simulink model "swapna_1"  (R2017a)
settings: Solver=VariableStepAuto  StartTime=0.0  StopTime=0.5  MaxStep=1e-4  RelTol=1e-3
libraries: powerlib x15
settings Model: Creator=Gali  LastModifiedBy=Gali

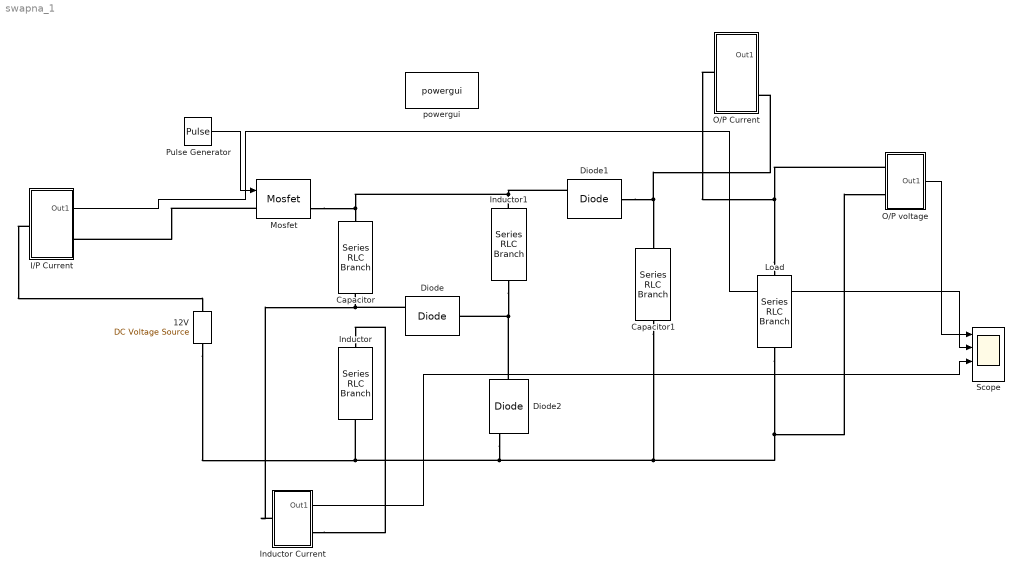
== system swapna_1 ==
  12V : powerlib/Electrical Sources/DC Voltage Source  Amplitude=12  Measurements=None
  Capacitor : powerlib/Elements/Series RLC Branch  LConnTagsString=__new0  RConnTagsString=__new0  BranchType=C  Resistance=1  Inductance=1e-3  SetiL0=off  InitialCurrent=0  Capacitance=47e-6  Setx0=off  InitialVoltage=0  Measurements=None
  Capacitor1 : powerlib/Elements/Series RLC Branch  LConnTagsString=__new0  RConnTagsString=__new0  BranchType=C  Resistance=1  Inductance=1e-3  SetiL0=off  InitialCurrent=0  Capacitance=270e-6  Setx0=off  InitialVoltage=0  Measurements=None
  Diode : powerlib/Power Electronics/Diode  Ron=0.001  Lon=0  Vf=0.8  IC=0  UseSnubber=0  Rs=500  Cs=250e-9  Measurements=on
  Diode1 : powerlib/Power Electronics/Diode  Ron=0.001  Lon=0  Vf=0.8  IC=0  UseSnubber=0  Rs=500  Cs=250e-9  Measurements=on
  Diode2 : powerlib/Power Electronics/Diode  Ron=0.001  Lon=0  Vf=0.8  IC=0  UseSnubber=0  Rs=500  Cs=250e-9  Measurements=on
  I/P Current : Subsystem
  Inductor : powerlib/Elements/Series RLC Branch  LConnTagsString=__new0  RConnTagsString=__new0  BranchType=L  Resistance=1  Inductance=1e-3  SetiL0=off  InitialCurrent=0  Capacitance=1e-6  Setx0=off  InitialVoltage=0  Measurements=None
  Inductor Current : Subsystem
  Inductor1 : powerlib/Elements/Series RLC Branch  LConnTagsString=__new0  RConnTagsString=__new0  BranchType=L  Resistance=1  Inductance=1e-3  SetiL0=off  InitialCurrent=0  Capacitance=1e-6  Setx0=off  InitialVoltage=0  Measurements=None
  Load : powerlib/Elements/Series RLC Branch  LConnTagsString=__new0  RConnTagsString=__new0  BranchType=R  Resistance=47  Inductance=1e-3  SetiL0=off  InitialCurrent=0  Capacitance=220e-6  Setx0=off  InitialVoltage=0  Measurements=None
  Mosfet : powerlib/Power Electronics/Mosfet  Ron=0.28  Lon=0  Rd=0.01  Vfd=0  IC=0  Rs=1e5  Cs=inf  Measurements=on
  O/P Current : Subsystem
  O/P voltage : Subsystem
  Pulse Generator : DiscretePulseGenerator  PulseType=Time based  Period=1/32000  PulseWidth=62.2
  Scope : Scope  NumInputPorts=4
  powergui : powerlib/powergui  Priority=1  SimulationMode=Continuous  SampleTime=50e-6  frequency=60  Iterations=50  frequencyindice=0  Pbase=100e6  ErrMax=1e-4  UnitsV=kV  UnitsW=MW  buscounter=0  FunctionMessages=off  echomessages=off  EnableUseOfTLC=off  CurrentSourceSwitches=off  DisableSnubberDevices=off  DisableRonSwitches=off  DisableVfSwitches=off  DisplayEquations=off  SolverType=Tustin/Backward Euler (TBE)  Interpol=off  ExternalGateDelay=off  methode=off  Ts=100  x0status=blocks  SPID=on  SwTol=0  HookPort=off  RestoreLinks=warning  ResistiveCurrentMeasurement=off  Frange=[0:2:500]  Ylog=off  Xlog=on  ShowGrid=off  save=off  variable=ZData  structure=0  ZoomFFT=off  StartTime=0.0  cycles=1  DisplayStyle=1  fundamental=60  FreqAxis=off  MaxFrequency=1000  frequencyindicesteady=1  RmsSteady=1  display=off
  wires:
  Pulse Generator/1 -> Mosfet/1
  I/P Current/1(Out1) -> Scope/2
  O/P voltage/1(Out1) -> Scope/1
  Inductor Current/1(Out1) -> Scope/3
  connections:
  Load/RConn1 -- O/P voltage/LConn2 -- Capacitor1/LConn1 -- Diode2/RConn1 -- 12V/LConn1 -- Inductor/RConn1
  Capacitor/RConn1 -- Diode1/RConn1 -- Inductor1/LConn1 -- Mosfet/RConn1
  Inductor1/RConn1 -- Diode2/LConn1 -- Diode/LConn1
  Diode1/LConn1 -- O/P Current/RConn1 -- Capacitor1/RConn1
  Mosfet/LConn1 -- I/P Current/RConn1
  I/P Current/LConn1 -- 12V/RConn1
  Load/LConn1 -- O/P voltage/LConn1 -- O/P Current/LConn1
  Capacitor/LConn1 -- Inductor Current/LConn1 -- Diode/RConn1
  Inductor Current/RConn1 -- Inductor/LConn1

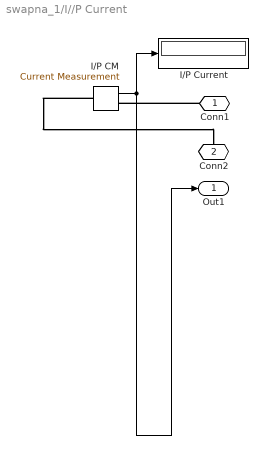
== system swapna_1/I//P Current ==
  I/P CM : powerlib/Measurements/Current Measurement  PhasorSimulation=off  OutputType=Complex  PSBequivalent=0
  I/P Current : Display
  Conn1 : PMIOPort  Port=1  Side=Right
  Conn2 : PMIOPort  Port=2  Side=Left
  Out1 : Outport
  wires:
  I/P CM/1 -> Out1/1, I/P Current/1
  connections:
  Conn1/RConn1 -- I/P CM/RConn1
  I/P CM/LConn1 -- Conn2/RConn1

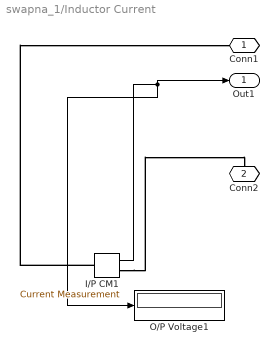
== system swapna_1/Inductor Current ==
  I/P CM1 : powerlib/Measurements/Current Measurement  PhasorSimulation=off  OutputType=Complex  PSBequivalent=0
  O/P Voltage1 : Display
  Conn1 : PMIOPort  Port=1  Side=Left
  Conn2 : PMIOPort  Port=2  Side=Right
  Out1 : Outport
  wires:
  I/P CM1/1 -> Out1/1, O/P Voltage1/1
  connections:
  I/P CM1/LConn1 -- Conn1/RConn1
  I/P CM1/RConn1 -- Conn2/RConn1

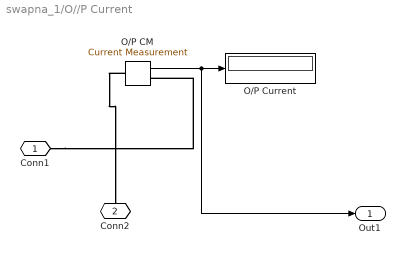
== system swapna_1/O//P Current ==
  O/P CM : powerlib/Measurements/Current Measurement  PhasorSimulation=off  OutputType=Complex  PSBequivalent=0
  O/P Current : Display
  Conn1 : PMIOPort  Port=1  Side=Right
  Conn2 : PMIOPort  Port=2  Side=Left
  Out1 : Outport
  wires:
  O/P CM/1 -> Out1/1, O/P Current/1
  connections:
  Conn1/RConn1 -- O/P CM/RConn1
  O/P CM/LConn1 -- Conn2/RConn1

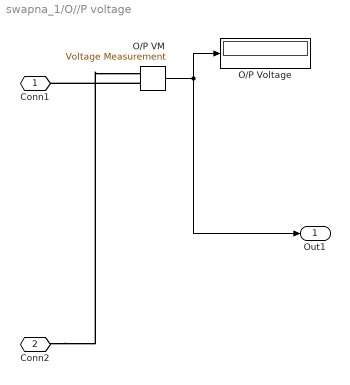
== system swapna_1/O//P voltage ==
  O/P VM : powerlib/Measurements/Voltage Measurement  PhasorSimulation=off  OutputType=Complex  PSBequivalent=0
  O/P Voltage : Display
  Conn1 : PMIOPort  Port=1  Side=Left
  Conn2 : PMIOPort  Port=2  Side=Left
  Out1 : Outport
  wires:
  O/P VM/1 -> Out1/1, O/P Voltage/1
  connections:
  Conn2/RConn1 -- O/P VM/LConn1
  O/P VM/LConn2 -- Conn1/RConn1
